simulink model "prison_rf_hybrid_kalman_model"  (R2024b)
settings: Solver=FixedStepDiscrete  StartTime=0.0  StopTime=116  FixedStep=1  RelTol=1e-3
settings Model: Creator=pnaga  LastModifiedBy=pnaga

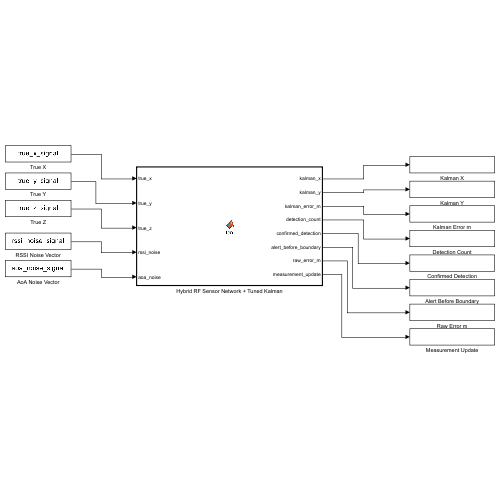
[thumbnail: Simulink's stored preview of the top-level diagram]
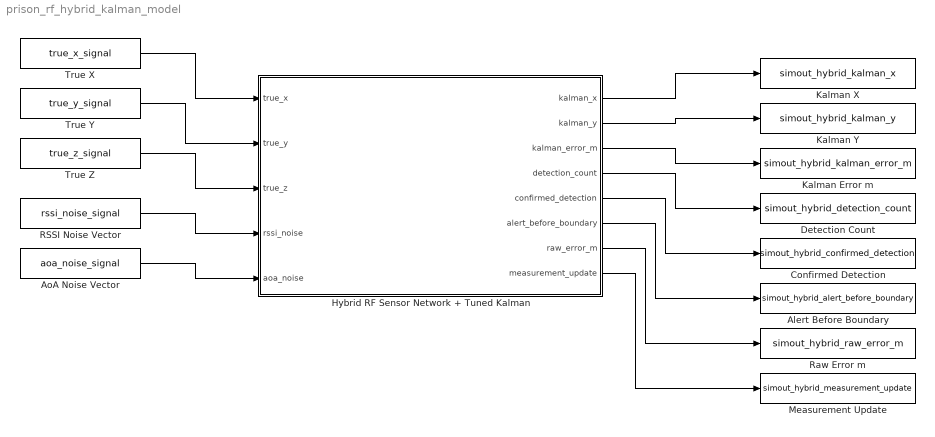
== system prison_rf_hybrid_kalman_model ==
  Alert Before Boundary : ToWorkspace  VariableName=simout_hybrid_alert_before_boundary  SaveFormat=Timeseries  SampleTime=-1
  AoA Noise Vector : FromWorkspace  VariableName=aoa_noise_signal
  Confirmed Detection : ToWorkspace  VariableName=simout_hybrid_confirmed_detection  SaveFormat=Timeseries  SampleTime=-1
  Detection Count : ToWorkspace  VariableName=simout_hybrid_detection_count  SaveFormat=Timeseries  SampleTime=-1
  Hybrid RF Sensor Network + Tuned Kalman : MATLAB Function  TreatAsAtomicUnit=on
  Kalman Error m : ToWorkspace  VariableName=simout_hybrid_kalman_error_m  SaveFormat=Timeseries  SampleTime=-1
  Kalman X : ToWorkspace  VariableName=simout_hybrid_kalman_x  SaveFormat=Timeseries  SampleTime=-1
  Kalman Y : ToWorkspace  VariableName=simout_hybrid_kalman_y  SaveFormat=Timeseries  SampleTime=-1
  Measurement Update : ToWorkspace  VariableName=simout_hybrid_measurement_update  SaveFormat=Timeseries  SampleTime=-1
  RSSI Noise Vector : FromWorkspace  VariableName=rssi_noise_signal
  Raw Error m : ToWorkspace  VariableName=simout_hybrid_raw_error_m  SaveFormat=Timeseries  SampleTime=-1
  True X : FromWorkspace  VariableName=true_x_signal
  True Y : FromWorkspace  VariableName=true_y_signal
  True Z : FromWorkspace  VariableName=true_z_signal
  wires:
  True X/1 -> Hybrid RF Sensor Network + Tuned Kalman/1(true_x)
  True Y/1 -> Hybrid RF Sensor Network + Tuned Kalman/2(true_y)
  True Z/1 -> Hybrid RF Sensor Network + Tuned Kalman/3(true_z)
  RSSI Noise Vector/1 -> Hybrid RF Sensor Network + Tuned Kalman/4(rssi_noise)
  AoA Noise Vector/1 -> Hybrid RF Sensor Network + Tuned Kalman/5(aoa_noise)
  Hybrid RF Sensor Network + Tuned Kalman/1(kalman_x) -> Kalman X/1
  Hybrid RF Sensor Network + Tuned Kalman/2(kalman_y) -> Kalman Y/1
  Hybrid RF Sensor Network + Tuned Kalman/3(kalman_error_m) -> Kalman Error m/1
  Hybrid RF Sensor Network + Tuned Kalman/4(detection_count) -> Detection Count/1
  Hybrid RF Sensor Network + Tuned Kalman/5(confirmed_detection) -> Confirmed Detection/1
  Hybrid RF Sensor Network + Tuned Kalman/6(alert_before_boundary) -> Alert Before Boundary/1
  Hybrid RF Sensor Network + Tuned Kalman/7(raw_error_m) -> Raw Error m/1
  Hybrid RF Sensor Network + Tuned Kalman/8(measurement_update) -> Measurement Update/1

== matlab function prison_rf_hybrid_kalman_model/Hybrid RF Sensor Network + Tuned Kalman ==
  data: true_x input double size=1; kalman_x output double size=1; true_y input double size=1; true_z input double size=1; rssi_noise input double size=24; aoa_noise input double size=24; kalman_y output double size=1; kalman_error_m output double size=1; detection_count output double size=1; confirmed_detection output double size=1; alert_before_boundary output double size=1; raw_error_m output double size=1; measurement_update output double size=1
function [kalman_x, kalman_y, kalman_error_m, detection_count, confirmed_detection, alert_before_boundary, raw_error_m, measurement_update] = hybridKalman(true_x, true_y, true_z, rssi_noise, aoa_noise)
%#codegen
persistent state P initialised last_x last_y
if isempty(initialised)
    state = zeros(4,1);
    P = diag([100 100 25 25]);
    initialised = false;
    last_x = true_x;
    last_y = true_y;
end
sensorX = [250;250;250;250;250;250;300;400;600;700;750;750;750;750;750;750;700;600;400;300;300;500;700;500];
sensorY = [300;350;450;550;650;700;700;700;700;700;700;650;550;450;350;300;300;300;300;300;500;350;500;650];
sensorZ = 15 * ones(24,1);
sensorType = [1;0;0;0;0;1;0;0;0;0;1;0;0;0;0;1;0;0;0;0;1;1;1;1];
orientation = atan2d(sensorY - 500, sensorX - 500);
fov = 120 * ones(24,1);
threshold = -70;
frequencyHz = 2.4e9;
txPowerDbm = 20;
rssiSigmaDb = 1;
aoaSigmaDeg = 0.5;
omniWeight = 0.02;
accelStd = 0.5;
measStd = 5;
gateM = 80;
rxNoisy = zeros(24,1);
measuredBearing = zeros(24,1);
detected = false(24,1);
detection_count = 0;
directional_count = 0;
for s = 1:24
    dx = true_x - sensorX(s);
    dy = true_y - sensorY(s);
    dz = true_z - sensorZ(s);
    distance = max(sqrt(dx*dx + dy*dy + dz*dz), 1);
    pathLossDb = 20*log10(distance) + 20*log10(frequencyHz) - 147.55;
    rxIdeal = txPowerDbm - pathLossDb;
    rxNoisy(s) = rxIdeal + rssi_noise(s);
    trueBearing = atan2d(dy, dx);
    if sensorType(s) == 1
        inFov = true;
        measuredBearing(s) = 0;
    else
        inFov = abs(wrap180Local(trueBearing - orientation(s))) <= fov(s)/2;
        measuredBearing(s) = wrap180Local(trueBearing + aoa_noise(s));
    end
    detected(s) = inFov && rxNoisy(s) >= threshold;
    if detected(s)
        detection_count = detection_count + 1;
        if sensorType(s) == 0
            directional_count = directional_count + 1;
        end
    end
end
confirmed_detection = double(detection_count >= 2);
outsideSecureWall = true_x < 300 || true_x > 700 || true_y < 350 || true_y > 650;
alert_before_boundary = double(confirmed_detection > 0 && outsideSecureWall);
raw_x = NaN; raw_y = NaN; raw_error_m = NaN;
if directional_count >= 2 || detection_count >= 3 || (directional_count >= 1 && detection_count >= 2)
    sensorXd = zeros(24,1); sensorYd = zeros(24,1); ranges = zeros(24,1); rangeStd = zeros(24,1); bearingRad = zeros(24,1); bearingMask = false(24,1); rangeScale = zeros(24,1);
    n = 0;
    for s = 1:24
        if detected(s)
            n = n + 1;
            sensorXd(n) = sensorX(s);
            sensorYd(n) = sensorY(s);
            ranges(n) = 10^((txPowerDbm - rxNoisy(s) - 20*log10(frequencyHz) + 147.55)/20);
            rangeStd(n) = max((log(10)/20) * rssiSigmaDb * ranges(n), 1);
            if sensorType(s) == 0
                bearingRad(n) = measuredBearing(s) * pi / 180;
                bearingMask(n) = true;
                rangeScale(n) = 1;
            else
                rangeScale(n) = omniWeight;
            end
        end
    end
    pos = [0;0]; countBearing = 0;
    for i = 1:n
        if bearingMask(i)
            countBearing = countBearing + 1;
            pos(1) = pos(1) + sensorXd(i) + ranges(i) * cos(bearingRad(i));
            pos(2) = pos(2) + sensorYd(i) + ranges(i) * sin(bearingRad(i));
        end
    end
    if countBearing > 0
        pos = pos / countBearing;
    else
        for i = 1:n
            pos(1) = pos(1) + sensorXd(i);
            pos(2) = pos(2) + sensorYd(i);
        end
        pos = pos / n;
    end
    bearingStd = aoaSigmaDeg*pi/180;
    for iter = 1:25
        Hmat = zeros(2,2); g = zeros(2,1);
        for i = 1:n
            dx = pos(1) - sensorXd(i);
            dy = pos(2) - sensorYd(i);
            predRange = max(sqrt(dx*dx + dy*dy), 1e-6);
            rr = predRange - ranges(i);
            Jr = [dx/predRange, dy/predRange];
            wr = rangeScale(i) / rangeStd(i);
            Hmat = Hmat + (Jr' * Jr) * wr * wr;
            g = g + Jr' * rr * wr * wr;
            if bearingMask(i)
                predBearing = atan2(dy, dx);
                rb = wrapPiLocal(predBearing - bearingRad(i));
                Jb = [-dy/(predRange*predRange), dx/(predRange*predRange)];
                wb = 1 / bearingStd;
                Hmat = Hmat + (Jb' * Jb) * wb * wb;
                g = g + Jb' * rb * wb * wb;
            end
        end
        step = -((Hmat + 1e-5*eye(2)) \ g);
        pos = pos + step;
        if sqrt(step(1)*step(1)+step(2)*step(2)) < 1e-4
            break;
        end
    end
    raw_x = pos(1); raw_y = pos(2);
    raw_error_m = sqrt((raw_x-true_x)^2 + (raw_y-true_y)^2);
end
dt = max(sqrt((true_x-last_x)^2 + (true_y-last_y)^2) / 15, 1);
if initialised
    F = [1 0 dt 0; 0 1 0 dt; 0 0 1 0; 0 0 0 1];
    q = accelStd^2;
    Q = q * [dt^4/4 0 dt^3/2 0; 0 dt^4/4 0 dt^3/2; dt^3/2 0 dt^2 0; 0 dt^3/2 0 dt^2];
    state = F * state;
    P = F * P * F' + Q;
end
measurement_update = 0;
if ~isnan(raw_x)
    z = [raw_x; raw_y];
    if ~initialised
        state = [raw_x; raw_y; 0; 0];
        initialised = true;
        measurement_update = 1;
    else
        Hk = [1 0 0 0; 0 1 0 0];
        R = (measStd^2) * eye(2);
        residual = z - Hk * state;
        if sqrt(residual(1)^2 + residual(2)^2) <= gateM
            Sk = Hk * P * Hk' + R;
            K = P * Hk' / Sk;
            state = state + K * residual;
            P = (eye(4) - K * Hk) * P;
            measurement_update = 1;
        end
    end
end
if initialised
    kalman_x = state(1);
    kalman_y = state(2);
    kalman_error_m = sqrt((kalman_x-true_x)^2 + (kalman_y-true_y)^2);
else
    kalman_x = NaN; kalman_y = NaN; kalman_error_m = NaN;
end
last_x = true_x; last_y = true_y;
end
function angle = wrap180Local(angle)
angle = mod(angle + 180, 360) - 180;
end
function angle = wrapPiLocal(angle)
angle = mod(angle + pi, 2*pi) - pi;
end
